simulink model "nonlin_feedback"  (R2023a)
settings: Solver=ode1  StartTime=0  StopTime=1200  FixedStep=0.002  RelTol=1e-3
values from neighbouring files (symbols this model uses):
  B1 = [-kQ, -kQ, kQ, kQ ... (first row only)    [advanced_model_setup.m]    (also in modelCompPlot.m; set_model_params.m)
  B2 = [0, 0, 0 ... (first row only)    [advanced_model_setup.m]    (also in modelCompPlot.m; set_model_params.m)
  cycleGain = 0.1    [advanced_model_setup.m]
  I_xx = 0.0522    [advanced_model_setup.m]    (also in modelCompPlot.m; set_model_params.m; solveSyms3d_2.m = evalin('base', 'I_xx'))
  I_yy = 0.0522    [advanced_model_setup.m]    (also in modelCompPlot.m; set_model_params.m; solveSyms3d_2.m = evalin('base', 'I_yy'))
  I_zz = 0.1104    [advanced_model_setup.m]    (also in modelCompPlot.m; set_model_params.m; solveSyms3d_2.m = evalin('base', 'I_zz'))
  K = K1    [advanced_model_setup.m]    (also in gainScheduling.m = lqi(sys, Q, R); lookupGainScheduling.m = gainScheduling([x1_range(n), x2_range(nn)]))
  k_T = 0.1188    [advanced_model_setup.m]    (also in modelCompPlot.m; set_model_params.m; solveSyms3d_2.m = evalin('base', 'k_T'))
  kd = 0.5    [advanced_model_setup.m]
  kfr_p = 0.4*u2line/x5line    (= 0.285774113641)    [advanced_model_setup.m]    (also in modelCompPlot.m; set_model_params.m)
  kfr_r = 0.4*u1line/x4line    (= 0.285774113641)    [advanced_model_setup.m]    (also in modelCompPlot.m; set_model_params.m)
  kfr_y = 0.4*u3line/x6line    (= 0.0880063173321)    [advanced_model_setup.m]    (also in modelCompPlot.m; set_model_params.m)
  l_a = 0.1968    [advanced_model_setup.m]    (also in modelCompPlot.m; set_model_params.m; solveSyms3d_2.m = evalin('base', 'l_a'))
  r = 0.2    [advanced_model_setup.m]    (also in gainScheduling.m = evalin('base', 'r'))
  sigma = 0    [modelCompPlot.m]
  skew = 1    [advanced_model_setup.m]
  V_bias = 12    [advanced_model_setup.m]    (also in modelCompPlot.m; set_model_params.m; solveSyms3d.m = evalin('base', 'V_bias'))
  VMAX_AMP = 24    [advanced_model_setup.m]    (also in modelCompPlot.m; set_model_params.m)
  wcf = 2 * pi * 20    (= 125.663706144)    [advanced_model_setup.m]    (also in modelCompPlot.m; set_model_params.m)
  zetaf = 0.6    [advanced_model_setup.m]    (also in modelCompPlot.m; set_model_params.m)
libraries: simulink_extras x4, dspsrcs4 x1
settings Model: Creator=kille  LastModifiedBy=Jacob

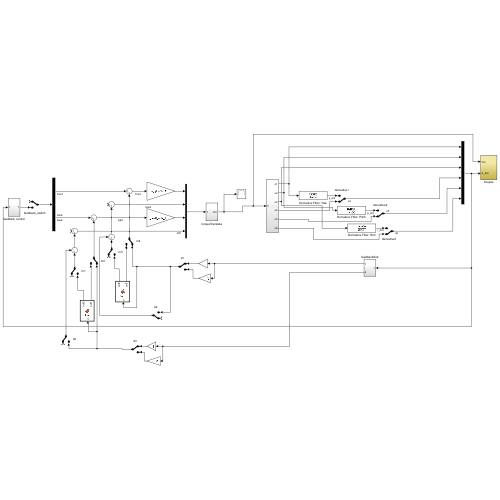
[thumbnail: Simulink's stored preview of the top-level diagram]
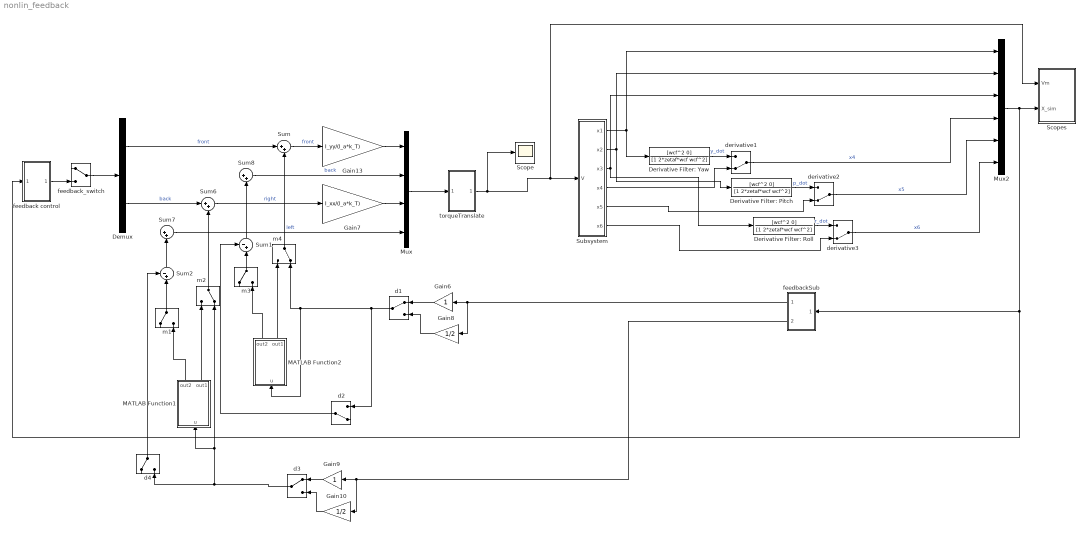
== system nonlin_feedback ==
  Demux : Demux  Outputs=2
  Derivative Filter: Pitch : TransferFcn  Numerator=[wcf^2 0]  Denominator=[1 2*zetaf*wcf wcf^2]
  Derivative Filter: Roll : TransferFcn  Numerator=[wcf^2 0]  Denominator=[1 2*zetaf*wcf wcf^2]
  Derivative Filter: Yaw : TransferFcn  Numerator=[wcf^2 0]  Denominator=[1 2*zetaf*wcf wcf^2]
  Gain10 : Gain  Gain=1/2
  Gain13 : Gain  Gain=I_yy/(l_a*k_T)
  Gain6 : Gain
  Gain7 : Gain  Gain=I_xx/(l_a*k_T)
  Gain8 : Gain  Gain=1/2
  Gain9 : Gain
  MATLAB Function1 : MATLAB Function  TreatAsAtomicUnit=on
  MATLAB Function2 : MATLAB Function  TreatAsAtomicUnit=on
  Mux : Mux
  Mux2 : Mux  Inputs=6
  Scope : Scope
  Scopes : Subsystem
  Subsystem : Subsystem
  Sum{,6..8} (4 alike) : Sum  Inputs=|++
  Sum1 : Sum  Inputs=-+|
  Sum2 : Sum  Inputs=-+|
  d1 : ManualSwitch
  d2 : ManualSwitch  CurrentSetting=0
  d3 : ManualSwitch
  d4 : ManualSwitch
  derivative1 : ManualSwitch  CurrentSetting=0
  derivative2 : ManualSwitch  CurrentSetting=0
  derivative3 : ManualSwitch  CurrentSetting=0
  feedback control : Subsystem
  feedbackSub : Subsystem
  feedback_switch : ManualSwitch
  m1 : ManualSwitch
  m2 : ManualSwitch  CurrentSetting=0
  m3 : ManualSwitch
  m4 : ManualSwitch  CurrentSetting=0
  torqueTranslate : Subsystem
  wires:
  d1/1 -> d2/1, MATLAB Function2/1(u), m4/2
  MATLAB Function2/1(out2) -> m3/2
  MATLAB Function1/2(out1) -> m2/1
  Sum7/1 -> Mux/4  "left"
  MATLAB Function1/1(out2) -> m1/2
  Sum/1 -> Gain13/1  "front"
  Demux/1 -> Sum/1  "front"
  Sum6/1 -> Gain7/1  "right"
  Sum8/1 -> Mux/2  "back"
  MATLAB Function2/2(out1) -> m4/1
  Derivative Filter: Yaw/1 -> derivative1/1  "y_dot"
  Derivative Filter: Pitch/1 -> derivative2/1  "p_dot"
  Derivative Filter: Roll/1 -> derivative3/1  "r_dot"
  Subsystem/1(x1) -> Mux2/1, Derivative Filter: Yaw/1
  Subsystem/4(x4) -> derivative1/2
  Subsystem/2(x2) -> Derivative Filter: Pitch/1, Mux2/2
  Subsystem/5(x5) -> derivative2/2
  Subsystem/6(x6) -> derivative3/2
  Subsystem/3(x3) -> Mux2/3, Derivative Filter: Roll/1
  m2/1 -> Sum6/2
  m4/1 -> Sum/2
  derivative3/1 -> Mux2/6  "x6"
  derivative2/1 -> Mux2/5  "x5"
  derivative1/1 -> Mux2/4  "x4"
  Gain6/1 -> d1/1
  Gain8/1 -> d1/2
  m3/1 -> Sum1/2
  Sum1/1 -> Sum8/2
  d2/1 -> Sum1/1
  Sum2/1 -> Sum7/2
  m1/1 -> Sum2/2
  Gain9/1 -> d3/1
  Gain10/1 -> d3/2
  d3/1 -> MATLAB Function1/1(u), m2/2, d4/2
  d4/1 -> Sum2/1
  feedbackSub/2(Out2) -> Gain10/1, Gain9/1
  feedbackSub/1(Out1) -> Gain8/1, Gain6/1
  Mux2/1 -> feedback control/1(In1), feedbackSub/1(Input), Scopes/2(X_sim)
  Demux/2 -> Sum6/1  "back"
  feedback_switch/1 -> Demux/1
  feedback control/1(Out1) -> feedback_switch/2
  Mux/1 -> torqueTranslate/1(In1)
  torqueTranslate/1(Vm) -> Scope/1, Scopes/1(Vm), Subsystem/1(V)
  Gain13/1 -> Mux/1
  Gain7/1 -> Mux/3

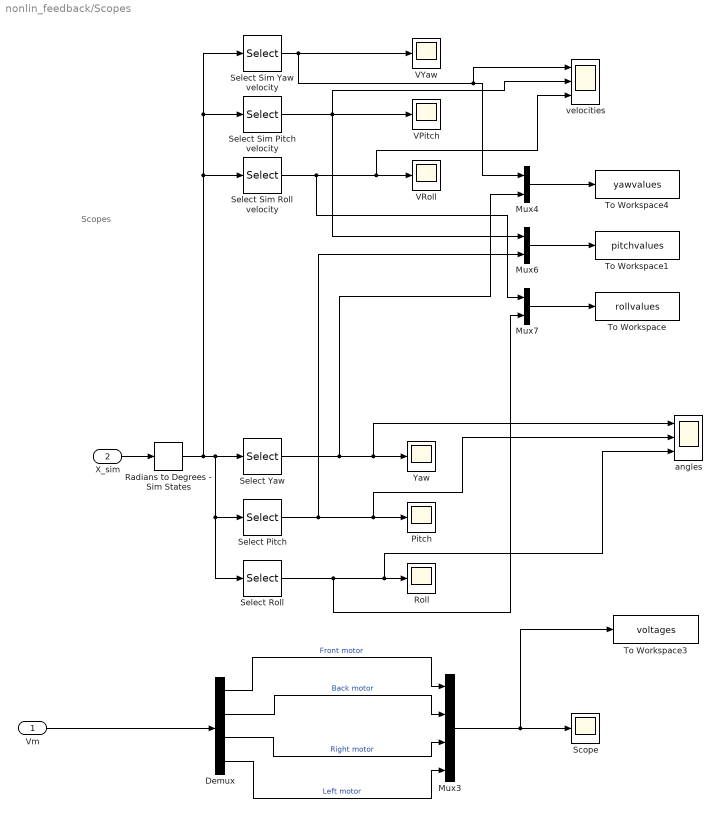
== system nonlin_feedback/Scopes ==
  note: Scopes
  Vm : Inport
  X_sim : Inport  Port=2
  Demux : Demux
  Mux3 : Mux
  Mux4 : Mux  Inputs=2
  Mux6 : Mux  Inputs=2
  Mux7 : Mux  Inputs=2
  Pitch : Scope
  Radians to Degrees - Sim States : simulink_extras/Transformations/Radians to Degrees
  Roll : Scope
  Scope : Scope
  Select Pitch : Selector  InputPortWidth=6  IndexOptions=Index vector (dialog)  Indices=2  OutputSizes=1
  Select Roll : Selector  InputPortWidth=6  IndexOptions=Index vector (dialog)  Indices=3  OutputSizes=1
  Select Sim Pitch velocity : Selector  InputPortWidth=6  IndexOptions=Index vector (dialog)  Indices=5  OutputSizes=1
  Select Sim Roll velocity : Selector  InputPortWidth=6  IndexOptions=Index vector (dialog)  Indices=6  OutputSizes=1
  Select Sim Yaw velocity : Selector  InputPortWidth=6  IndexOptions=Index vector (dialog)  Indices=4  OutputSizes=1
  Select Yaw : Selector  InputPortWidth=6  IndexOptions=Index vector (dialog)  Indices=1  OutputSizes=1
  To Workspace : ToWorkspace  VariableName=rollvalues  SampleTime=-1
  To Workspace1 : ToWorkspace  VariableName=pitchvalues  SampleTime=-1
  To Workspace3 : ToWorkspace  VariableName=voltages  SampleTime=-1
  To Workspace4 : ToWorkspace  VariableName=yawvalues  SampleTime=-1
  VPitch : Scope
  VRoll : Scope
  VYaw : Scope
  Yaw : Scope
  angles : Scope  NumInputPorts=3
  velocities : Scope  NumInputPorts=3
  wires:
  Select Roll/1 -> angles/3, Roll/1, Mux7/2
  Radians to Degrees - Sim States/1 -> Select Sim Roll velocity/1, Select Sim Pitch velocity/1, Select Sim Yaw velocity/1, Select Roll/1, Select Pitch/1, Select Yaw/1
  Select Pitch/1 -> angles/2, Pitch/1, Mux6/2
  X_sim/1 -> Radians to Degrees - Sim States/1
  Demux/1 -> Mux3/1  "Front motor"
  Demux/2 -> Mux3/2  "Back motor"
  Demux/3 -> Mux3/3  "Right motor"
  Demux/4 -> Mux3/4  "Left motor"
  Vm/1 -> Demux/1
  Select Sim Yaw velocity/1 -> VYaw/1, velocities/1, Mux4/1
  Select Sim Roll velocity/1 -> velocities/3, VRoll/1, Mux7/1
  Select Sim Pitch velocity/1 -> Mux6/1, velocities/2, VPitch/1
  Mux4/1 -> To Workspace4/1
  Mux6/1 -> To Workspace1/1
  Mux7/1 -> To Workspace/1
  Mux3/1 -> To Workspace3/1, Scope/1
  Select Yaw/1 -> angles/1, Yaw/1, Mux4/2

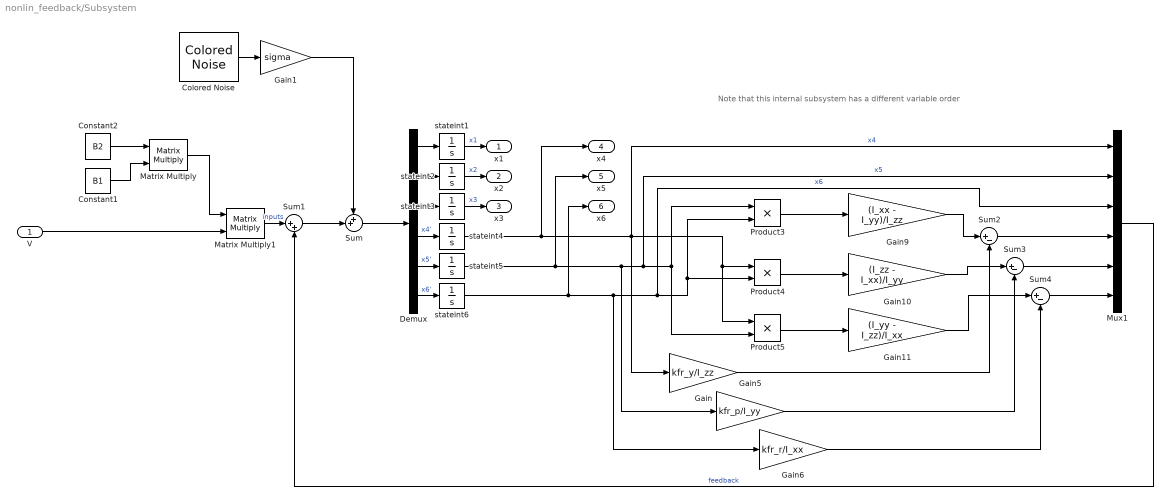
== system nonlin_feedback/Subsystem ==
  note: Note that this internal subsystem has a different variable order
  V : Inport
  Colored Noise : dspsrcs4/Colored Noise  Color=white  InverseFrequencyPower=1  BoundedOutput=off  NumChannels=6  OutputDataType=double  SamplesPerFrame=1  SampleTime=1  RandomStream=mt19937ar with seed  Seed=67  SimulateUsing=Interpreted execution
  Constant1 : Constant  Value=B1
  Constant2 : Constant  Value=B2
  Demux : Demux  Outputs=6
  Gain : Gain  Gain=kfr_y/I_zz
  Gain1 : Gain  Gain=sigma
  Gain10 : Gain  Gain=(I_zz - I_xx)/I_yy
  Gain11 : Gain  Gain=(I_yy - I_zz)/I_xx
  Gain5 : Gain  Gain=kfr_p/I_yy
  Gain6 : Gain  Gain=kfr_r/I_xx
  Gain9 : Gain  Gain=(I_xx - I_yy)/I_zz
  Matrix Multiply : Product  Multiplication=Matrix(*)
  Matrix Multiply1 : Product  Multiplication=Matrix(*)
  Mux1 : Mux  Inputs=6
  Product3 : Product
  Product4 : Product
  Product5 : Product
  Sum : Sum  Inputs=++|
  Sum1 : Sum  Inputs=|++
  Sum2 : Sum  Inputs=|+-
  Sum3 : Sum  Inputs=|+-
  Sum4 : Sum  Inputs=|+-
  stateint1 : Integrator  InitialCondition=0.017453
  stateint2 : Integrator  InitialCondition=0.017453
  stateint3 : Integrator  InitialCondition=0.017453
  stateint4 : Integrator
  stateint5 : Integrator
  stateint6 : Integrator
  x1 : Outport
  x2 : Outport  Port=2
  x3 : Outport  Port=3
  x4 : Outport  Port=4
  x5 : Outport  Port=5
  x6 : Outport  Port=6
  wires:
  Mux1/1 -> Sum1/2  "feedback"
  stateint5/1 -> x5/1, Gain5/1, Mux1/2, Product5/2, Product3/1  "x5"
  Matrix Multiply1/1 -> Sum1/1  "inputs"
  stateint4/1 -> x4/1, Gain/1, Mux1/1, Product5/1, Product4/1  "x4"
  Matrix Multiply/1 -> Matrix Multiply1/1
  V/1 -> Matrix Multiply1/2
  Sum2/1 -> Mux1/4
  Gain6/1 -> Sum4/2
  Demux/1 -> stateint1/1
  stateint6/1 -> x6/1, Gain6/1, Mux1/3, Product4/2, Product3/2  "x6"
  Demux/6 -> stateint6/1  "x6'"
  Product5/1 -> Gain11/1
  Demux/5 -> stateint5/1  "x5'"
  Demux/2 -> stateint2/1
  Gain11/1 -> Sum4/1
  Constant1/1 -> Matrix Multiply/2
  Demux/3 -> stateint3/1
  Gain9/1 -> Sum2/1
  Gain10/1 -> Sum3/1
  Constant2/1 -> Matrix Multiply/1
  Demux/4 -> stateint4/1  "x4'"
  Product4/1 -> Gain10/1
  stateint1/1 -> x1/1  "x1"
  stateint2/1 -> x2/1  "x2"
  stateint3/1 -> x3/1  "x3"
  Colored Noise/1 -> Gain1/1
  Sum1/1 -> Sum/2
  Sum/1 -> Demux/1
  Gain1/1 -> Sum/1
  Product3/1 -> Gain9/1
  Gain/1 -> Sum2/2
  Gain5/1 -> Sum3/2
  Sum4/1 -> Mux1/6
  Sum3/1 -> Mux1/5

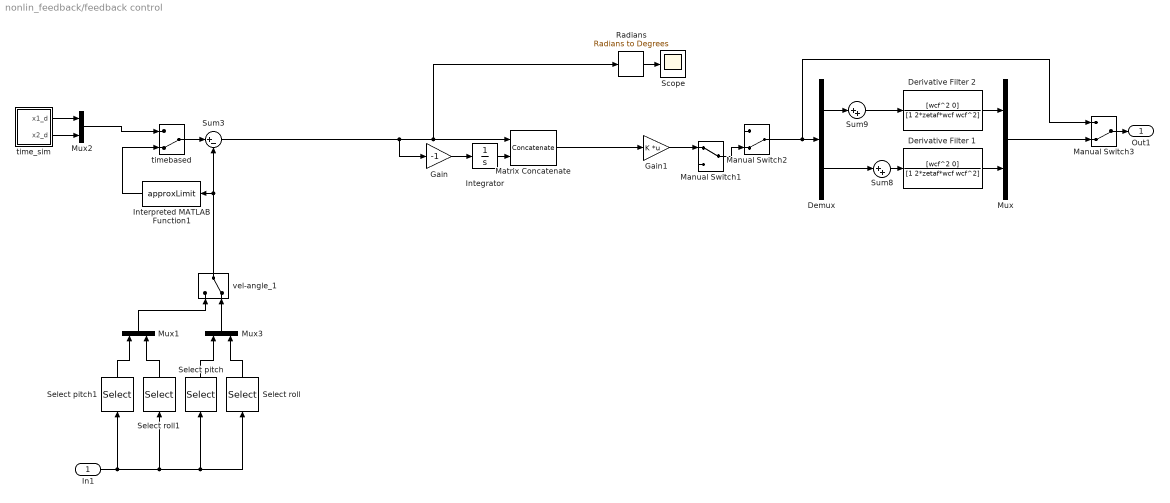
== system nonlin_feedback/feedback control ==
  In1 : Inport
  Demux : Demux  Outputs=2
  Derivative Filter 1 : TransferFcn  Numerator=[wcf^2 0]  Denominator=[1 2*zetaf*wcf wcf^2]
  Derivative Filter 2 : TransferFcn  Numerator=[wcf^2 0]  Denominator=[1 2*zetaf*wcf wcf^2]
  Gain : Gain  Gain=-1
  Gain1 : Gain  Gain=K  Multiplication=Matrix(K*u)
  Integrator : Integrator
  Interpreted MATLAB Function1 : MATLABFcn  MATLABFcn=approxLimit  Output1D=off
  Manual Switch1 : ManualSwitch
  Manual Switch2 : ManualSwitch  CurrentSetting=0
  Manual Switch3 : ManualSwitch  CurrentSetting=0
  Matrix Concatenate : Concatenate  Mode=Multidimensional array
  Mux{,1..3} (4 alike) : Mux  Inputs=2
  Radians : simulink_extras/Transformations/Radians to Degrees
  Scope : Scope
  Select pitch : Selector  InputPortWidth=6  IndexOptions=Index vector (dialog)  Indices=2  OutputSizes=1
  Select pitch1 : Selector  InputPortWidth=6  IndexOptions=Index vector (dialog)  Indices=5  OutputSizes=1
  Select roll : Selector  InputPortWidth=6  IndexOptions=Index vector (dialog)  Indices=3  OutputSizes=1
  Select roll1 : Selector  InputPortWidth=6  IndexOptions=Index vector (dialog)  Indices=6  OutputSizes=1
  Sum3 : Sum  Inputs=|+-
  Sum8 : Sum  Inputs=|++
  Sum9 : Sum  Inputs=|++
  time_sim : Subsystem
  timebased : ManualSwitch  CurrentSetting=0
  vel-angle_1 : ManualSwitch  CurrentSetting=0
  Out1 : Outport
  wires:
  time_sim/1(x1_d) -> Mux2/1
  time_sim/2(x2_d) -> Mux2/2
  Mux3/1 -> vel-angle_1/2
  Select roll1/1 -> Mux1/2
  Select pitch1/1 -> Mux1/1
  Mux1/1 -> vel-angle_1/1
  Select roll/1 -> Mux3/2
  In1/1 -> Select roll1/1, Select roll/1, Select pitch/1, Select pitch1/1
  Select pitch/1 -> Mux3/1
  Demux/1 -> Sum9/1
  Derivative Filter 2/1 -> Mux/1
  Sum9/1 -> Derivative Filter 2/1
  Manual Switch3/1 -> Out1/1
  Derivative Filter 1/1 -> Mux/2
  Demux/2 -> Sum8/1
  Sum8/1 -> Derivative Filter 1/1
  Mux/1 -> Manual Switch3/2
  Manual Switch2/1 -> Manual Switch3/1, Demux/1
  Interpreted MATLAB Function1/1 -> timebased/2
  vel-angle_1/1 -> Sum3/2, Interpreted MATLAB Function1/1
  Mux2/1 -> timebased/1
  timebased/1 -> Sum3/1
  Radians/1 -> Scope/1
  Sum3/1 -> Gain/1, Radians/1, Matrix Concatenate/1
  Gain1/1 -> Manual Switch1/1
  Integrator/1 -> Matrix Concatenate/2
  Matrix Concatenate/1 -> Gain1/1
  Gain/1 -> Integrator/1
  Manual Switch1/1 -> Manual Switch2/2

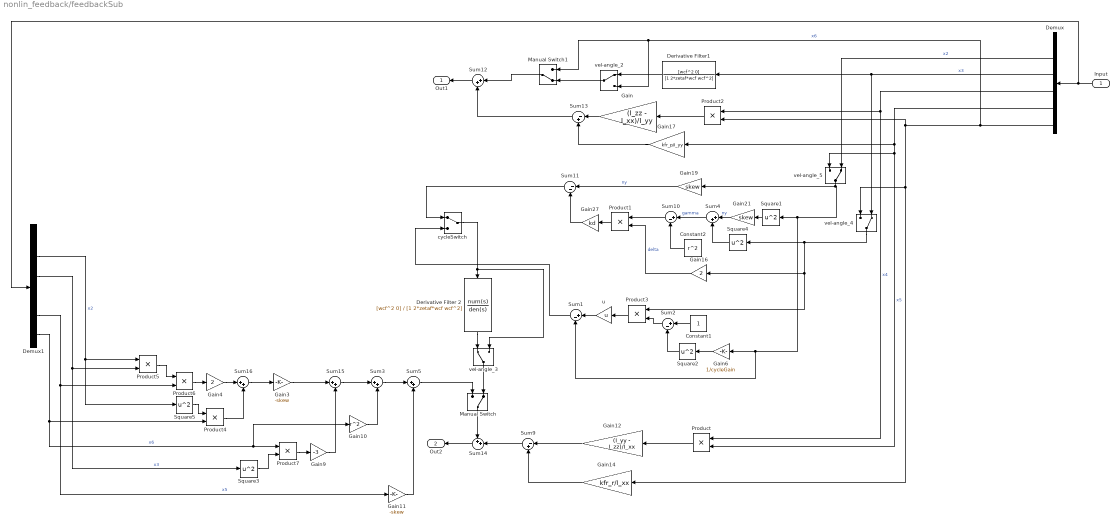
== system nonlin_feedback/feedbackSub ==
  Input : Inport
  Constant1 : Constant
  Constant2 : Constant  Value=r^2
  Demux : Demux  Outputs=6
  Demux1 : Demux  Outputs=6
  Derivative Filter 2 : TransferFcn  Numerator=[wcf^2 0]  Denominator=[1 2*zetaf*wcf wcf^2]
  Derivative Filter1 : TransferFcn  Numerator=[wcf^2 0]  Denominator=[1 2*zetaf*wcf wcf^2]
  Gain : Gain  Gain=(I_zz - I_xx)/I_yy
  Gain10 : Gain  Gain=r^2
  Gain11 : Gain  Gain=-skew
  Gain12 : Gain  Gain=(I_yy - I_zz)/I_xx
  Gain14 : Gain  Gain=kfr_r/I_xx
  Gain16 : Gain  Gain=2
  Gain17 : Gain  Gain=kfr_p/I_yy
  Gain19 : Gain  Gain=skew
  Gain21 : Gain  Gain=skew
  Gain27 : Gain  Gain=kd
  Gain3 : Gain  Gain=-skew
  Gain4 : Gain  Gain=2
  Gain6 : Gain  Gain=1/cycleGain
  Gain9 : Gain  Gain=-3
  Manual Switch : ManualSwitch  CurrentSetting=0
  Manual Switch1 : ManualSwitch  CurrentSetting=0
  Product{,1..7} (8 alike) : Product
  Square{1..5} (5 alike) : Math  Operator=square
  Sum1 : Sum  Inputs=|+-
  Sum10 : Sum  Inputs=|+-
  Sum11 : Sum  Inputs=|--
  Sum{3..5,12,15..16} (6 alike) : Sum  Inputs=|++
  Sum13 : Sum  Inputs=|-+
  Sum14 : Sum  Inputs=++|
  Sum2 : Sum  Inputs=|+-
  Sum9 : Sum  Inputs=|-+
  cycleSwitch : ManualSwitch
  u : Gain  Gain=u
  vel-angle_2 : ManualSwitch
  vel-angle_3 : ManualSwitch
  vel-angle_4 : ManualSwitch  CurrentSetting=0
  vel-angle_5 : ManualSwitch  CurrentSetting=0
  Out1 : Outport
  Out2 : Outport  Port=2
  wires:
  Derivative Filter1/1 -> vel-angle_2/1
  Gain17/1 -> Sum13/2
  Sum13/1 -> Sum12/2
  Demux/4 -> Product/1, Product2/1  "x4"
  Gain21/1 -> Sum4/1  "ny"
  Product2/1 -> Gain/1
  Demux/5 -> vel-angle_5/1, Product/2, Gain17/1  "x5"
  Gain27/1 -> Sum11/2
  Product/1 -> Gain12/1
  Constant2/1 -> Sum10/2
  Sum10/1 -> Product1/1
  Demux/6 -> vel-angle_2/2, Manual Switch1/1, vel-angle_4/1, Gain14/1, Product2/2  "x6"
  Sum4/1 -> Sum10/1  "gamma"
  Sum9/1 -> Sum14/2
  Square4/1 -> Sum4/2
  Gain12/1 -> Sum9/1
  Square1/1 -> Gain21/1
  Product1/1 -> Gain27/1
  Gain/1 -> Sum13/1
  Gain14/1 -> Sum9/2
  Sum12/1 -> Out1/1
  Gain19/1 -> Sum11/1  "ny"
  Gain16/1 -> Product1/2  "delta"
  Sum14/1 -> Out2/1
  Square2/1 -> Sum2/2
  Demux/2 -> vel-angle_5/2  "x2"
  Constant1/1 -> Sum2/1
  Sum2/1 -> Product3/2
  Product3/1 -> u/1
  Gain6/1 -> Square2/1
  Demux/3 -> vel-angle_4/2, Derivative Filter1/1  "x3"
  u/1 -> Sum1/1
  Sum11/1 -> cycleSwitch/1
  cycleSwitch/1 -> vel-angle_3/2, Derivative Filter 2/1
  Sum1/1 -> cycleSwitch/2
  vel-angle_4/1 -> Square4/1, Product3/1, Gain16/1
  vel-angle_5/1 -> Gain6/1, Sum1/2, Square1/1, Gain19/1
  Derivative Filter 2/1 -> vel-angle_3/1
  Input/1 -> Demux1/1, Demux/1
  Demux1/2 -> Product5/1, Square5/1  "x2"
  Demux1/5 -> Gain11/1, Product6/2  "x5"
  Product7/1 -> Gain9/1
  Sum3/1 -> Sum5/1
  Demux1/6 -> Gain10/1, Product7/1, Product4/2  "x6"
  Gain3/1 -> Sum15/1
  Sum15/1 -> Sum3/1
  Square5/1 -> Product4/1
  Product5/1 -> Product6/1
  Gain11/1 -> Sum5/2
  Gain4/1 -> Sum16/1
  Gain10/1 -> Sum3/2
  Square3/1 -> Product7/2
  Product4/1 -> Sum16/2
  Product6/1 -> Gain4/1
  Gain9/1 -> Sum15/2
  Sum16/1 -> Gain3/1
  Demux1/3 -> Square3/1, Product5/2  "x3"
  Manual Switch/1 -> Sum14/1
  vel-angle_3/1 -> Manual Switch/2
  Sum5/1 -> Manual Switch/1
  vel-angle_2/1 -> Manual Switch1/2
  Manual Switch1/1 -> Sum12/1

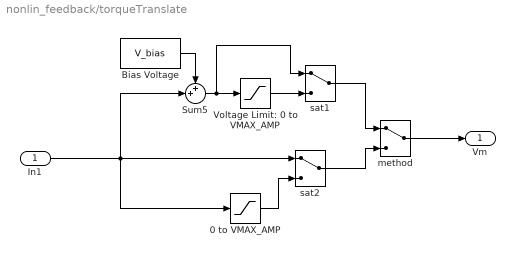
== system nonlin_feedback/torqueTranslate ==
  In1 : Inport
  0 to VMAX_AMP : Saturate  UpperLimit=VMAX_AMP  LowerLimit=0
  Bias Voltage : Constant  Value=V_bias
  Sum5 : Sum  Inputs=++|
  Voltage Limit: 0 to VMAX_AMP : Saturate  UpperLimit=VMAX_AMP  LowerLimit=0
  method : ManualSwitch  Tag=swt
  sat1 : ManualSwitch
  sat2 : ManualSwitch
  Vm : Outport
  wires:
  Sum5/1 -> sat1/1, Voltage Limit: 0 to VMAX_AMP/1
  Bias Voltage/1 -> Sum5/1
  Voltage Limit: 0 to VMAX_AMP/1 -> sat1/2
  0 to VMAX_AMP/1 -> sat2/2
  sat1/1 -> method/1
  method/1 -> Vm/1
  sat2/1 -> method/2
  In1/1 -> 0 to VMAX_AMP/1, sat2/1, Sum5/2

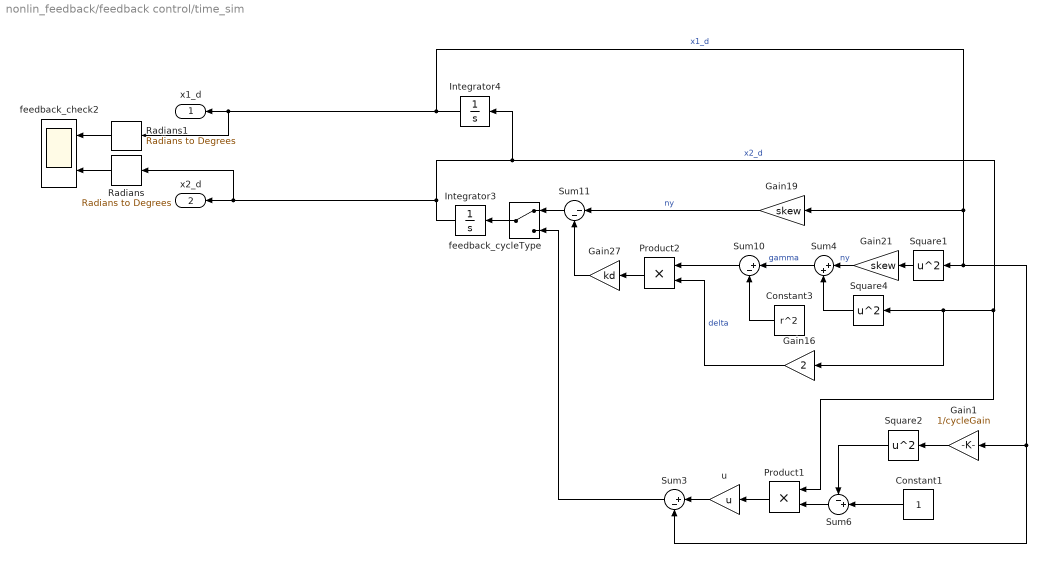
== system nonlin_feedback/feedback control/time_sim ==
  Constant1 : Constant
  Constant3 : Constant  Value=r^2
  Gain1 : Gain  Gain=1/cycleGain
  Gain16 : Gain  Gain=2
  Gain19 : Gain  Gain=skew
  Gain21 : Gain  Gain=skew
  Gain27 : Gain  Gain=kd
  Integrator3 : Integrator  InitialCondition=0.00010472
  Integrator4 : Integrator  InitialCondition=0.00010472
  Product1 : Product
  Product2 : Product
  Radians : simulink_extras/Transformations/Radians to Degrees
  Radians1 : simulink_extras/Transformations/Radians to Degrees
  Square1 : Math  Operator=square
  Square2 : Math  Operator=square
  Square4 : Math  Operator=square
  Sum10 : Sum  Inputs=|+-
  Sum11 : Sum  Inputs=|--
  Sum3 : Sum  Inputs=|+-
  Sum4 : Sum  Inputs=|++
  Sum6 : Sum  Inputs=-+|
  feedback_check2 : Scope  NumInputPorts=2
  feedback_cycleType : ManualSwitch
  u : Gain  Gain=u
  x1_d : Outport
  x2_d : Outport  Port=2
  wires:
  Square1/1 -> Gain21/1
  Square4/1 -> Sum4/2
  Integrator4/1 -> Sum3/2, Gain1/1, Square1/1, Gain19/1, Radians1/1, x1_d/1  "x1_d"
  Gain27/1 -> Sum11/2
  Gain16/1 -> Product2/2  "delta"
  Gain19/1 -> Sum11/1  "ny"
  Integrator3/1 -> Product1/1, Gain16/1, Square4/1, Integrator4/1, Radians/1, x2_d/1  "x2_d"
  Sum10/1 -> Product2/1
  Constant3/1 -> Sum10/2
  Gain21/1 -> Sum4/1  "ny"
  Sum4/1 -> Sum10/1  "gamma"
  Product2/1 -> Gain27/1
  Radians1/1 -> feedback_check2/1
  Radians/1 -> feedback_check2/2
  Square2/1 -> Sum6/1
  Gain1/1 -> Square2/1
  u/1 -> Sum3/1
  Product1/1 -> u/1
  Sum6/1 -> Product1/2
  Constant1/1 -> Sum6/2
  feedback_cycleType/1 -> Integrator3/1
  Sum11/1 -> feedback_cycleType/1
  Sum3/1 -> feedback_cycleType/2

== matlab function nonlin_feedback/MATLAB Function2 ==
  data: out2 output; u input; out1 output
function [out2, out1] = fcn(u)

if u > 0
    out1 = u;
    out2 = 0;
else
    out1 = 0;
    out2 = -u;
end

== matlab function nonlin_feedback/MATLAB Function1 ==
  data: out2 output; u input; out1 output
function [out2, out1] = fcn(u)

if u > 0
    out1 = u;
    out2 = 0;
else
    out1 = 0;
    out2 = -u;
end
